simulink model "servopositioner"  (R2013a)
settings: Solver=ode45  StartTime=0.0  StopTime=10.0  RelTol=1e-3
model workspace (MATLAB code in the model file):
  | % Data obtained from:
  | % ------------------------------------------------------------
  | % HyQ-Robot: Standard Definition for Joint Angles
  | % and Kinematic Parameters of the Legs and Torso
  | %
  | % Project: HyQ-Robot V1.0 with Leg V2.0
  | % Genoa, 9th July 2010
  | %-------------------------------------------------------------
  | % This Matlab file was made by:
  | % Job Ledezma
  | % Genova, Feb 2016
  | %-------------------------------------------------------------
  | 
  | 
  | % ________________________________________
  | %
  | %                HYL DESCRIPTION PARAMETERS
  | %________________________________________
  | 
  | % ---- Leg data ------
  | 
  | m1 = 1.772;              % Kg - Upper leg mass
  | m2 = 0.808;              % Kg - Lower leg mass
  | M = 3.982;                % Kg - Base mass
  | P_01 = 0.08;             % m - distance P0-P1
  | P_12 = 0.350;           % m - distance P1-P2
  | P_23 = 0.330;           % m - distance P2-P3
  | FR = 0.02;                 % m - foot radius
  | P1m1 = 0.164;           % m - distance P1-Pm1
  | P2m2 = 0.122;           % m - distance P2-Pm2
  | I1zz = 0.0713;           % kg·m2 - Inertia upper leg
  | I2zz = 0.0218;           % kg·m2 - Inertia lower leg
  | em1 = deg2rad(7.9);  % rad
  | em2 = deg2rad(0);     % rad
  | g  = 9.810;                 % m/s2 - gravity
  | 
  | % ----- Lever Arm Parameters -----
  | 
  | % Hip joint
  | a1   = 0.3219;             % m
  | b1   = 0.045;               % m
  | e11 = deg2rad(6.24); % rad
  | e12 = deg2rad(0);      % rad
  | 
  | % Knee joint
  | a2 = 0.3218;               % m
  | b2 = 0.045;                 % m
  | e21 = deg2rad(8.04);  % rad
  | e22 = deg2rad(6);       % rad
  | 
  | % ----- Limit Angles --------
  | 
  | % Initial conditions
  | q0_0 = 1;                           % m - height of the floating base
  | q1_0 = deg2rad(45);         % rad - HFE angle
  | q2_0 = deg2rad(-90);        % rad - KFE angle
  | 
  | % Max angle limits
  | q1Max = deg2rad(70);       % rad
  | q2Max = deg2rad(-20);      % rad
  | 
  | % Min angle limits
  | q1Min = deg2rad(-50);        % rad
  | q2Min = deg2rad(-140);      % rad
  | q0Min = P_01+P_12*cos(q1Min)+P_23*cos(q1Min+q2Min)+FR;     % m
  | 
  | % ________________________________________________________
  | %
  | %                                        HYDRAULIC PARAMETERS
  | % ________________________________________________________
  | 
  | % ------ Power unit --------
  | 
  | ps  = 160e5;                            % Pa - Supply pressure
  | pt  = 10e5;                              % Pa - Tank pressure
  | dpt = ps - pt;                           % Pa - Delta pressure
  | beta = 1.4e9;                          % Pa- Effective bulk modulus
  | 
  | % Initial condition for integrators
  | xo = 0;
  | 
  | pAo = 0;%ps/2;
  | pBo = 0;%ps/2;
  | 
  | %----- Cylinder - HOERBIGER LB6 16 10 0080 4M ----------
  | 
  | Dp = 0.016;                             % m - Piston diameter
  | Dr = 0.010;                              % m - Rod diameter
  | L  = 0.080;                               % m- Stroke
  | Aa = pi*(Dp^2)/4;                   % m^2 - Area A of the piston
  | Ab = pi*(Dp^2-Dr^2)/4;         % m^2 - Area B of the piston
  | r  = Aa/Ab;                              % Relation between areas
  | fv = 700;                                 %  Ns/m - Viscous friction
  | leak =1.7*10^-13;                 % m3/(s.Pa) - Cylinder leakage
  | Mp = ((pi*Dr^2/4)*L + Aa*0.15)*7860;    % Kg - Piston mass (approximated)
  | Lcyl = 0.280;                           % m - Total length of the cylinder
  | 
  | %-----  Valve Parameters - MOOG E024 - 177LA ----------
  | 
  | In   = 10;                               % I - Nominal control current
  | Qn   = 7.5 / 60e3;                 % m^3/s - Nominal flow rate
  | dptn = 70e5;                         % Pa - Valve pressure drop
  | Qlk   = 0.375 / 60e3;               % m^3/s - Leakage flow
  | Plk    = 70e5;                       % Pa - Nominal supply pressure for leakage test
  | wn    = 2*100*pi;                    % rad/s - Valve's natural frequency
  | E       = 0.7;                           % Valve's damping coefficient
  | Kv     = Qn/sqrt(dptn);          % m^3/(s*sqrt(Pa)) - Total flow coefficient
  | Kva    = Kv*sqrt(2);               % m^3/(s*sqrt(Pa)) - Partial flow coefficient A
  | Kvb    = Kv*sqrt(2);               % m^3/(s*sqrt(Pa)) - Partial flow coefficient B
  | Kvlk   = Qlk/sqrt(2*Plk);         % m^3/(s*sqrt(Pa)) - Total leakage flow coefficient
  | KvlkA  = Kvlk;                         % m^3/(s*sqrt(Pa)) -  Partial leakage flow coefficient A
  | KvlkB  = Kvlk;                         % m^3/(s*sqrt(Pa)) - Partial leakage flow coefficient B
  | up_dz = 0;                             % V - Upper limit of dead zone
  | lw_dz = 0;                              % V - Lower limit of dead zone
  | 
  | %------------   Manifold  -----------
  | % Review this part with the manifold's CAD design
  | 
  | v1a = (pi*(0.0035^2)/4)*0.07255;
  | v2a = (pi*(0.006^2)/4)*(0.090-0.012);
  | v1b = (pi*(0.0035^2)/4)*0.04491;
  | v2b = (pi*(0.006^2)/4)*(0.019+0.009);
  | v3b = (pi*(0.006^2)/4)*(0.007+0.009);
  | V0A = v1a + v2a;                                            % Dead volume coupled to chamber A
  | V0B = v1b + v2b + v3b;                                  % Dead volume coupled to chamber B
  | 
  | %-------  Load cell - BURSTER 8417-6005 ----------
  | 
  | xs = 20e-6;                            % m - Maximum deflection @ full scale
  | Fs = 5000;                             % N - Maximum force
  | Ks = Fs / xs ;                         % N·m - Load cell stiffness
  | 
  | noise = 0;                            %N - noise due nonlinearities, hysteresis, non repeatibility
  | 
  | %------ Accumulator - FOX-ITALY HST 0,04 ----------
  | 
  | acc = 0;
  | 
  | n = 1.4;                                % Polytropic constant
  | V0 = 0.04e-3;                       % m3 - Initial volume
  | P0 = 100e5 + 1e5;               % Pa - Precharge pressure
libraries: simulink x1
settings Model: Creator=Toshiba  LastModifiedBy=Toshiba

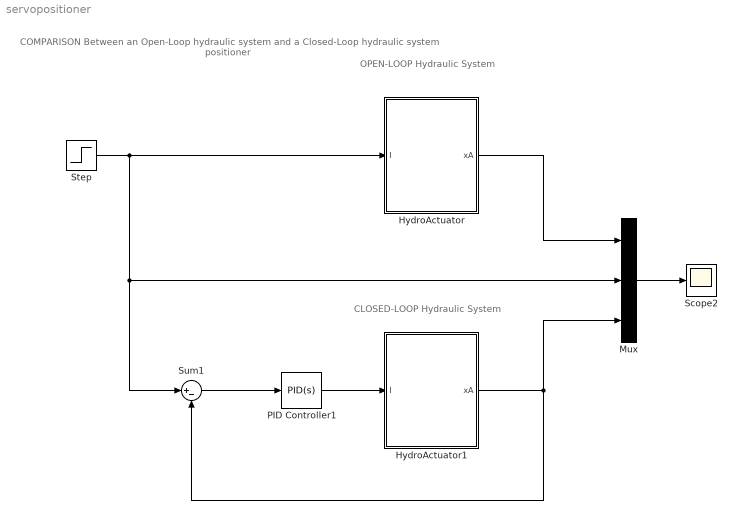
== system servopositioner ==
  note: OPEN-LOOP
      | Hydraulic System
  note: COMPARISON Between
      | an Open-Loop hydraulic system
      | and a Closed-Loop hydraulic
      | system positioner
  note: CLOSED-LOOP
      | Hydraulic System
  HydroActuator : Subsystem
  HydroActuator1 : Subsystem
  Mux : Mux  Inputs=3
  PID Controller1 : simulink/Continuous/PID Controller  Controller=PID  TimeDomain=Continuous-time  SampleTime=1  IntegratorMethod=Forward Euler  FilterMethod=Forward Euler  Form=Parallel  P=400  I=50  D=0  N=100  InitialConditionSource=internal  InitialConditionForIntegrator=0  InitialConditionForFilter=0  ExternalReset=none  LimitOutput=off  UpperSaturationLimit=inf  LowerSaturationLimit=-inf  LinearizeAsGain=on  AntiWindupMode=none  Kb=1  TrackingMode=off  Kt=1  PParamMin=[]  PParamMax=[]  IParamMin=[]  IParamMax=[]  DParamMin=[]  DParamMax=[]  NParamMin=[]  NParamMax=[]  KbParamMin=[]  KbParamMax=[]  KtParamMin=[]  KtParamMax=[]  POutMin=[]  POutMax=[]  IOutMin=[]  IOutMax=[]  DOutMin=[]  DOutMax=[]  NOutMin=[]  NOutMax=[]  KbOutMin=[]  KbOutMax=[]  KtOutMin=[]  KtOutMax=[]  IntegratorOutMin=[]  IntegratorOutMax=[]  FilterOutMin=[]  FilterOutMax=[]  SumOutMin=[]  SumOutMax=[]  SumI1OutMin=[]  SumI1OutMax=[]  SumI2OutMin=[]  SumI2OutMax=[]  SumI3OutMin=[]  SumI3OutMax=[]  SumDOutMin=[]  SumDOutMax=[]  SaturationOutMin=[]  SaturationOutMax=[]  IntegratorContinuousStateAttributes=''  IntegratorStateMustResolveToSignalObject=off  IntegratorRTWStateStorageClass=Auto  FilterContinuousStateAttributes=''  FilterStateMustResolveToSignalObject=off  FilterRTWStateStorageClass=Auto
  Scope2 : Scope
      settings: YMin=-152500  YMax=-117500
  Step : Step  Time=3  After=0.04  SampleTime=0
  Sum1 : Sum  Inputs=|+-
  wires:
  Step/1 -> Mux/2, Sum1/1, HydroActuator/1(I)
  PID Controller1/1 -> HydroActuator1/1(I)
  HydroActuator/1(xA) -> Mux/1
  Mux/1 -> Scope2/1
  HydroActuator1/1(xA) -> Mux/3, Sum1/2
  Sum1/1 -> PID Controller1/1

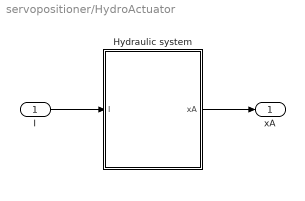
== system servopositioner/HydroActuator ==
  I : Inport
  Hydraulic system : Subsystem
  xA : Outport
  wires:
  I/1 -> Hydraulic system/1(I)
  Hydraulic system/1(xA) -> xA/1

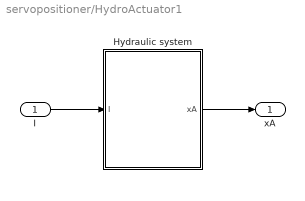
== system servopositioner/HydroActuator1 ==
  I : Inport
  Hydraulic system : Subsystem
  xA : Outport
  wires:
  Hydraulic system/1(xA) -> xA/1
  I/1 -> Hydraulic system/1(I)

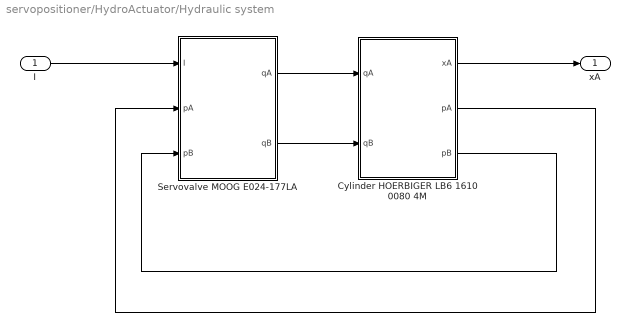
== system servopositioner/HydroActuator/Hydraulic system ==
  I : Inport
  Cylinder HOERBIGER LB6 1610 0080 4M : Subsystem
  Servovalve MOOG E024-177LA : Subsystem
  xA : Outport
  wires:
  Servovalve MOOG E024-177LA/2(qB) -> Cylinder HOERBIGER LB6 1610 0080 4M/2(qB)
  Servovalve MOOG E024-177LA/1(qA) -> Cylinder HOERBIGER LB6 1610 0080 4M/1(qA)
  Cylinder HOERBIGER LB6 1610 0080 4M/2(pA) -> Servovalve MOOG E024-177LA/2(pA)
  Cylinder HOERBIGER LB6 1610 0080 4M/3(pB) -> Servovalve MOOG E024-177LA/3(pB)
  I/1 -> Servovalve MOOG E024-177LA/1(I)
  Cylinder HOERBIGER LB6 1610 0080 4M/1(xA) -> xA/1

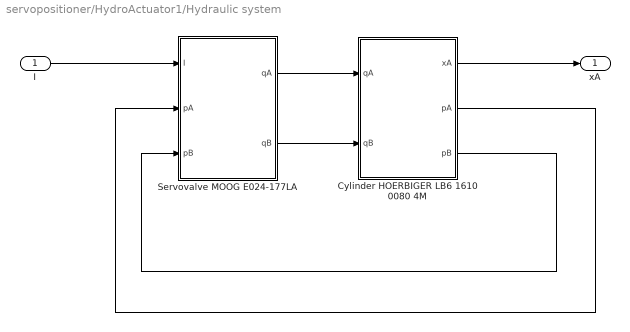
== system servopositioner/HydroActuator1/Hydraulic system ==
  I : Inport
  Cylinder HOERBIGER LB6 1610 0080 4M : Subsystem
  Servovalve MOOG E024-177LA : Subsystem
  xA : Outport
  wires:
  Cylinder HOERBIGER LB6 1610 0080 4M/1(xA) -> xA/1
  I/1 -> Servovalve MOOG E024-177LA/1(I)
  Cylinder HOERBIGER LB6 1610 0080 4M/3(pB) -> Servovalve MOOG E024-177LA/3(pB)
  Cylinder HOERBIGER LB6 1610 0080 4M/2(pA) -> Servovalve MOOG E024-177LA/2(pA)
  Servovalve MOOG E024-177LA/1(qA) -> Cylinder HOERBIGER LB6 1610 0080 4M/1(qA)
  Servovalve MOOG E024-177LA/2(qB) -> Cylinder HOERBIGER LB6 1610 0080 4M/2(qB)

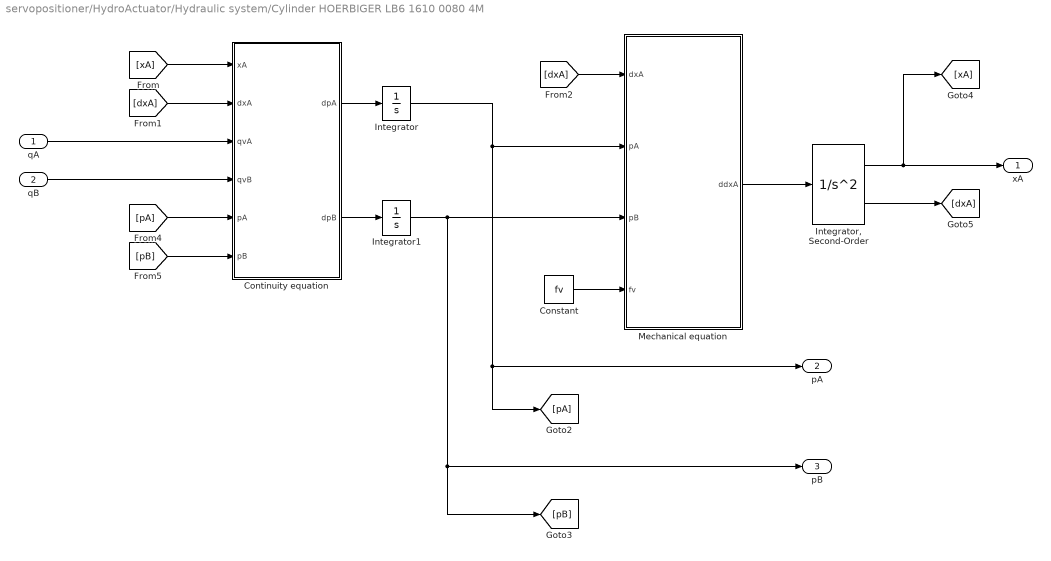
== system servopositioner/HydroActuator/Hydraulic system/Cylinder HOERBIGER LB6 1610 0080 4M ==
  qA : Inport
  qB : Inport  Port=2
  Constant : Constant  Value=fv
  Continuity equation : MATLAB Function  TreatAsAtomicUnit=on
  Integrator : Integrator  InitialCondition=pAo
  "Integrator, Second-Order" : SecondOrderIntegrator  ICX=xo  LimitX=on  UpperLimitX=L  LowerLimitX=0
  Integrator1 : Integrator  InitialCondition=pBo
  Mechanical equation : MATLAB Function  TreatAsAtomicUnit=on
  xA : Outport
  pA : Outport  Port=2
  pB : Outport  Port=3
  wires:
  Continuity equation/1(dpA) -> Integrator/1
  Continuity equation/2(dpB) -> Integrator1/1
  qA/1 -> Continuity equation/3(qvA)
  qB/1 -> Continuity equation/4(qvB)
  [dxA] -> Continuity equation/2(dxA)
  [xA] -> Continuity equation/1(xA)
  Constant/1 -> Mechanical equation/4(fv)
  [dxA] -> Mechanical equation/1(dxA)
  Integrator/1 -> [pA], pA/1, Mechanical equation/2(pA)
  Integrator1/1 -> [pB], pB/1, Mechanical equation/3(pB)
  [pA] -> Continuity equation/5(pA)
  [pB] -> Continuity equation/6(pB)
  Mechanical equation/1(ddxA) -> "Integrator, Second-Order"/1
  "Integrator, Second-Order"/1 -> xA/1, [xA]
  "Integrator, Second-Order"/2 -> [dxA]

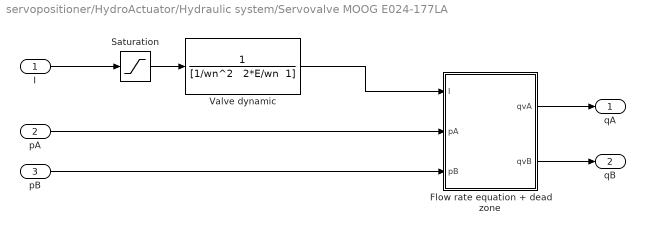
== system servopositioner/HydroActuator/Hydraulic system/Servovalve MOOG E024-177LA ==
  I : Inport
  pA : Inport  Port=2
  pB : Inport  Port=3
  Flow rate equation + dead zone : MATLAB Function  TreatAsAtomicUnit=on
  Saturation : Saturate  UpperLimit=In  LowerLimit=-In  LinearizeAsGain=off
  Valve dynamic : TransferFcn  Numerator=1  Denominator="[1/wn^2   2*E/wn  1]"
  qA : Outport
  qB : Outport  Port=2
  wires:
  Saturation/1 -> Valve dynamic/1
  I/1 -> Saturation/1
  Valve dynamic/1 -> Flow rate equation + dead zone/1(I)
  pA/1 -> Flow rate equation + dead zone/2(pA)
  pB/1 -> Flow rate equation + dead zone/3(pB)
  Flow rate equation + dead zone/2(qvB) -> qB/1
  Flow rate equation + dead zone/1(qvA) -> qA/1

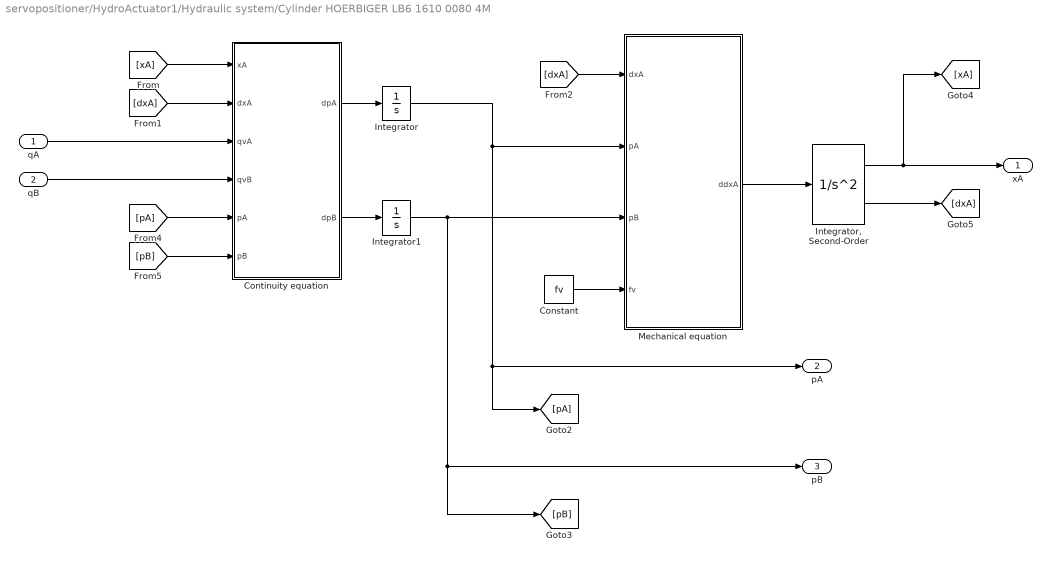
== system servopositioner/HydroActuator1/Hydraulic system/Cylinder HOERBIGER LB6 1610 0080 4M ==
  qA : Inport
  qB : Inport  Port=2
  Constant : Constant  Value=fv
  Continuity equation : MATLAB Function  TreatAsAtomicUnit=on
  Integrator : Integrator  InitialCondition=pAo
  "Integrator, Second-Order" : SecondOrderIntegrator  ICX=xo  LimitX=on  UpperLimitX=L  LowerLimitX=0
  Integrator1 : Integrator  InitialCondition=pBo
  Mechanical equation : MATLAB Function  TreatAsAtomicUnit=on
  xA : Outport
  pA : Outport  Port=2
  pB : Outport  Port=3
  wires:
  "Integrator, Second-Order"/2 -> [dxA]
  "Integrator, Second-Order"/1 -> [xA], xA/1
  Mechanical equation/1(ddxA) -> "Integrator, Second-Order"/1
  [pB] -> Continuity equation/6(pB)
  [pA] -> Continuity equation/5(pA)
  Integrator1/1 -> Mechanical equation/3(pB), pB/1, [pB]
  Integrator/1 -> Mechanical equation/2(pA), pA/1, [pA]
  [dxA] -> Mechanical equation/1(dxA)
  Constant/1 -> Mechanical equation/4(fv)
  [xA] -> Continuity equation/1(xA)
  [dxA] -> Continuity equation/2(dxA)
  qB/1 -> Continuity equation/4(qvB)
  qA/1 -> Continuity equation/3(qvA)
  Continuity equation/2(dpB) -> Integrator1/1
  Continuity equation/1(dpA) -> Integrator/1

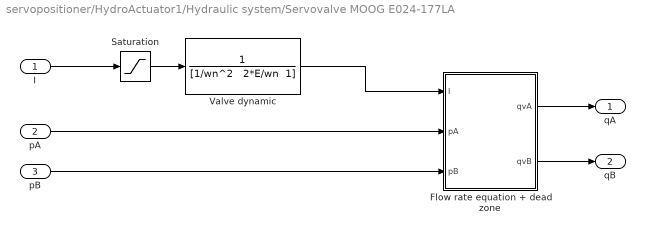
== system servopositioner/HydroActuator1/Hydraulic system/Servovalve MOOG E024-177LA ==
  I : Inport
  pA : Inport  Port=2
  pB : Inport  Port=3
  Flow rate equation + dead zone : MATLAB Function  TreatAsAtomicUnit=on
  Saturation : Saturate  UpperLimit=In  LowerLimit=-In  LinearizeAsGain=off
  Valve dynamic : TransferFcn  Numerator=1  Denominator="[1/wn^2   2*E/wn  1]"
  qA : Outport
  qB : Outport  Port=2
  wires:
  Flow rate equation + dead zone/1(qvA) -> qA/1
  Flow rate equation + dead zone/2(qvB) -> qB/1
  pB/1 -> Flow rate equation + dead zone/3(pB)
  pA/1 -> Flow rate equation + dead zone/2(pA)
  Valve dynamic/1 -> Flow rate equation + dead zone/1(I)
  I/1 -> Saturation/1
  Saturation/1 -> Valve dynamic/1

== matlab function servopositioner/HydroActuator1/Hydraulic system/Cylinder HOERBIGER LB6 1610 0080 4M/Continuity equation ==
  data: xA input; dpA output; dpB output; dxA input; qvA input; qvB input; pA input; pB input; leak parameter; V0A parameter; V0B parameter; Aa parameter; Ab parameter; L parameter; beta parameter; n parameter; V0 parameter; P0 parameter; acc parameter
function [dpA,dpB] = fcn(xA, dxA, qvA, qvB, pA, pB, leak, V0A, V0B, Aa, Ab, L, beta, n, V0, P0, acc)

pC = pA - pB;   % Pressao de carga [Pa]

qvlk = leak * pC;
dpa = 0;
dpb = 0;

if acc == 0,
%       /              \
%       |     beta     | /                    \
% dpA = | ------------ | | qvA - Aa*dx - qvex | 
%       |  Va0 + Aa*x  | \                    /
%       \              /
      
dpa = (beta/(V0A + Aa*xA)) * (qvA - Aa*dxA - qvlk);

%       /                  \
%       |     beta         | /                    \
% dpB = | ---------------- | | Ab*dx + qvex - qvB | 
%       | Vb0 + Ab*(L - x) | \                    /
%       \                  /
      
dpb = (beta/(V0B + Ab*(L-xA))) * (Ab*dxA + qvlk - qvB);

elseif acc == 1,
    
CA_A  = (V0A + Aa*xA) / beta;                      % Capacitancia hidráulica do atuador [m^3/Pa]
CAC_A = (V0*P0^(1/n))/(n* (pA+1e5)^((n+1)/n));     % Capacitancia hidráulica do acumulador [m^3/Pa]
CA_B  = (V0B + Ab*(L-xA)) / beta;                  % Capacitancia hidráulica do atuador [m^3/Pa]
CAC_B = (V0*P0^(1/n))/(n* (pB+1e5)^((n+1)/n));     % Capacitancia hidráulica do acumulador [m^3/Pa]

CT_A  = CA_A + CAC_A;                              % Capacitancia total em A
CT_B  = CA_B + CAC_B;                              % Capacitancia total em B 


%       /        \
%       |   1    | /                    \
% dpA = | ------ | | qvA - Aa*dx - qvex | 
%       |  CT_A  | \                    /
%       \        /
      
dpa = CT_A^-1 * (qvA - Aa*dxA - qvlk);

%       /        \
%       |   1    | /                    \
% dpB = | ------ | | Ab*dx + qvex - qvB | 
%       |  CT_B  | \                    /
%       \        /
      
dpb = CT_B^-1 * (Ab*dxA + qvlk - qvB);
end

dpA = dpa;
dpB = dpb;

== matlab function servopositioner/HydroActuator1/Hydraulic system/Cylinder HOERBIGER LB6 1610 0080 4M/Mechanical equation ==
  data: ddxA output; dxA input; pA input; pB input; fv input; Aa parameter; Ab parameter; Mp parameter
function ddxA = fcn(dxA, pA, pB, fv, Aa, Ab, Mp)
%#codegen

FH  = pA*Aa - pB*Ab;     % N - Hydraulic force
Ffr = fv*dxA;            % N - Friction force (Viscous)
ddxA  = (FH - Ffr)/Mp;     % m/s2 - Acceleration

== matlab function servopositioner/HydroActuator/Hydraulic system/Cylinder HOERBIGER LB6 1610 0080 4M/Continuity equation ==
  data: xA input; dpA output; dpB output; dxA input; qvA input; qvB input; pA input; pB input; leak parameter; V0A parameter; V0B parameter; Aa parameter; Ab parameter; L parameter; beta parameter; n parameter; V0 parameter; P0 parameter; acc parameter
function [dpA,dpB] = fcn(xA, dxA, qvA, qvB, pA, pB, leak, V0A, V0B, Aa, Ab, L, beta, n, V0, P0, acc)

pC = pA - pB;   % Pressao de carga [Pa]

qvlk = leak * pC;
dpa = 0;
dpb = 0;

if acc == 0,
%       /              \
%       |     beta     | /                    \
% dpA = | ------------ | | qvA - Aa*dx - qvex | 
%       |  Va0 + Aa*x  | \                    /
%       \              /
      
dpa = (beta/(V0A + Aa*xA)) * (qvA - Aa*dxA - qvlk);

%       /                  \
%       |     beta         | /                    \
% dpB = | ---------------- | | Ab*dx + qvex - qvB | 
%       | Vb0 + Ab*(L - x) | \                    /
%       \                  /
      
dpb = (beta/(V0B + Ab*(L-xA))) * (Ab*dxA + qvlk - qvB);

elseif acc == 1,
    
CA_A  = (V0A + Aa*xA) / beta;                      % Capacitancia hidráulica do atuador [m^3/Pa]
CAC_A = (V0*P0^(1/n))/(n* (pA+1e5)^((n+1)/n));     % Capacitancia hidráulica do acumulador [m^3/Pa]
CA_B  = (V0B + Ab*(L-xA)) / beta;                  % Capacitancia hidráulica do atuador [m^3/Pa]
CAC_B = (V0*P0^(1/n))/(n* (pB+1e5)^((n+1)/n));     % Capacitancia hidráulica do acumulador [m^3/Pa]

CT_A  = CA_A + CAC_A;                              % Capacitancia total em A
CT_B  = CA_B + CAC_B;                              % Capacitancia total em B 


%       /        \
%       |   1    | /                    \
% dpA = | ------ | | qvA - Aa*dx - qvex | 
%       |  CT_A  | \                    /
%       \        /
      
dpa = CT_A^-1 * (qvA - Aa*dxA - qvlk);

%       /        \
%       |   1    | /                    \
% dpB = | ------ | | Ab*dx + qvex - qvB | 
%       |  CT_B  | \                    /
%       \        /
      
dpb = CT_B^-1 * (Ab*dxA + qvlk - qvB);
end

dpA = dpa;
dpB = dpb;

== matlab function servopositioner/HydroActuator/Hydraulic system/Cylinder HOERBIGER LB6 1610 0080 4M/Mechanical equation ==
  data: ddxA output; dxA input; pA input; pB input; fv input; Aa parameter; Ab parameter; Mp parameter
function ddxA = fcn(dxA, pA, pB, fv, Aa, Ab, Mp)
%#codegen

FH  = pA*Aa - pB*Ab;     % N - Hydraulic force
Ffr = fv*dxA;            % N - Friction force (Viscous)
ddxA  = (FH - Ffr)/Mp;     % m/s2 - Acceleration

== matlab function servopositioner/HydroActuator1/Hydraulic system/Servovalve MOOG E024-177LA/Flow rate equation + dead zone ==
  data I settings: updateMethod=SF_CONTINUOUS_TIME_DATA
  data qvA settings: updateMethod=SF_CONTINUOUS_TIME_DATA
  data qvB settings: updateMethod=SF_CONTINUOUS_TIME_DATA
  data: I input; qvA output; qvB output; In parameter; Kva parameter; Kvb parameter; KvlkA parameter; KvlkB parameter; up_dz parameter; lw_dz parameter; ps parameter; pt parameter; pA input; pB input
function [qvA , qvB] = fcn(I, In, Kva, Kvb, KvlkA, KvlkB,up_dz, lw_dz, ps, pt, pA, pB)

if (I>=up_dz) && (I<=In),
    qvA = (Kva*(I/In) + KvlkA) * sign(ps-pA)*sqrt(abs(ps-pA)) - KvlkA*sign(pA-pt)*sqrt(abs(pA-pt)) ;
    qvB = (Kvb*(I/In) + KvlkB) * sign(pB-pt)*sqrt(abs(pB-pt)) - KvlkB*sign(ps-pB)*sqrt(abs(ps-pB)) ;
elseif (I>=-In) && (I<=lw_dz), 
    qvA = KvlkA*sign(ps-pA)*sqrt(abs(ps-pA)) - (Kva*(abs(I)/In) + KvlkA) * sign(pA-pt)*sqrt(abs(pA-pt));
     qvB = KvlkB*sign(pB-pt)*sqrt(abs(pB-pt)) - (Kvb*(abs(I)/In) + KvlkB) * sign(ps-pB)*sqrt(abs(ps-pB));
else
    qvA = 0;
    qvB = 0;
end
end

== matlab function servopositioner/HydroActuator/Hydraulic system/Servovalve MOOG E024-177LA/Flow rate equation + dead zone ==
  data I settings: updateMethod=SF_CONTINUOUS_TIME_DATA
  data qvA settings: updateMethod=SF_CONTINUOUS_TIME_DATA
  data qvB settings: updateMethod=SF_CONTINUOUS_TIME_DATA
  data: I input; qvA output; qvB output; In parameter; Kva parameter; Kvb parameter; KvlkA parameter; KvlkB parameter; up_dz parameter; lw_dz parameter; ps parameter; pt parameter; pA input; pB input
function [qvA , qvB] = fcn(I, In, Kva, Kvb, KvlkA, KvlkB,up_dz, lw_dz, ps, pt, pA, pB)

if (I>=up_dz) && (I<=In),
    qvA = (Kva*(I/In) + KvlkA) * sign(ps-pA)*sqrt(abs(ps-pA)) - KvlkA*sign(pA-pt)*sqrt(abs(pA-pt)) ;
    qvB = (Kvb*(I/In) + KvlkB) * sign(pB-pt)*sqrt(abs(pB-pt)) - KvlkB*sign(ps-pB)*sqrt(abs(ps-pB)) ;
elseif (I>=-In) && (I<=lw_dz), 
    qvA = KvlkA*sign(ps-pA)*sqrt(abs(ps-pA)) - (Kva*(abs(I)/In) + KvlkA) * sign(pA-pt)*sqrt(abs(pA-pt));
     qvB = KvlkB*sign(pB-pt)*sqrt(abs(pB-pt)) - (Kvb*(abs(I)/In) + KvlkB) * sign(ps-pB)*sqrt(abs(ps-pB));
else
    qvA = 0;
    qvB = 0;
end
end
